simulink model "WischerBox"  (R2017b)
settings: Solver=FixedStepAuto  StartTime=0.0  StopTime=10.0  RelTol=1e-3
PreLoadFcn:
  | waijung.modelPreload; % Required for working with Waijung Blockset. Do not remove.
undefined symbols (not defined in the file): Blocking, HSEOSC, Link, LQFP100, Non, Raw, ST, STM32F407VG
libraries: simulink x16, stm32f4_canbus_lib x5, stm32f4_io_lib x2, stm32f4_adc_lib x1, stm32f4_device_config_lib x1
CloseFcn:
  | waijung.modelClose; % Required for working with Waijung Blockset. Do not remove.
settings Model: Creator=labuser  LastModifiedBy=labuser
settings OptimizationCC: DefaultParameterBehavior=Inlined  PassReuseOutputArgsAs=Individual arguments
settings DebuggingCC: ParameterTunabilityLossMsg=error
settings HardwareCC: ProdBitPerPointer=32  ProdBitPerSizeT=32  ProdBitPerPtrDiffT=32  ProdLargestAtomicFloat=None  ProdIntDivRoundTo=Undefined  ProdWordSize=32  ProdHWDeviceType=ARM Compatible->Cortex - M4  TargetEndianess=LittleEndian  TargetHWDeviceType=ARM Compatible->Cortex - M4
settings SFSimCC: MATLABDynamicMemAlloc=off
settings RTWCC: SystemTargetFile=stm32f4.tlc  GenerateMakefile=off  TemplateMakefile=ert_default_tmf  Description=STM32F4 Target  GenerateReport=on  IncludeHyperlinkInReport=on  LaunchReport=on  GenerateTraceInfo=on  GenerateTraceReport=on  GenerateTraceReportSl=on  GenerateTraceReportSf=on  GenerateTraceReportEml=on
settings CodeAppCC: ForceParamTrailComments=on  IgnoreCustomStorageClasses=off  OperatorAnnotations=on  SimulinkDataObjDesc=on  SFDataObjDesc=on  InsertBlockDesc=on
settings STFCustomTargetCC: TargetLangStandard=C99 (ISO)  MultiwordLength=256  ModelReferenceCompliant=off  CombineOutputUpdateFcns=on  ERTCustomFileBanners=on  SupportContinuousTime=off  SupportNonInlinedSFcns=off  RemoveResetFunc=on  MATLABClassNameForMDSCustomization=Simulink.SoftwareTarget.ERTCustomization  GRTInterface=off  SystemTargetFile=stm32f4.tlc
settings ERTTargetCC: TargetLangStandard=C99 (ISO)  ModelReferenceCompliant=off  ParMdlRefBuildCompliant=off  CompOptLevelCompliant=off  ConcurrentExecutionCompliant=off  ModelStepFunctionPrototypeControlCompliant=off  CPPClassGenCompliant=off  UseToolchainInfoCompliant=off  InlinedParameterPlacement=NonHierarchical  ERTSrcFileBannerTemplate=stm32f4_code_template.cgt  ERTHdrFileBannerTemplate=stm32f4_code_template.cgt  ERTDataSrcFileTemplate=stm32f4_code_template.cgt  ERTDataHdrFileTemplate=stm32f4_code_template.cgt  ERTCustomFileTemplate=stm32f4_file_process.tlc

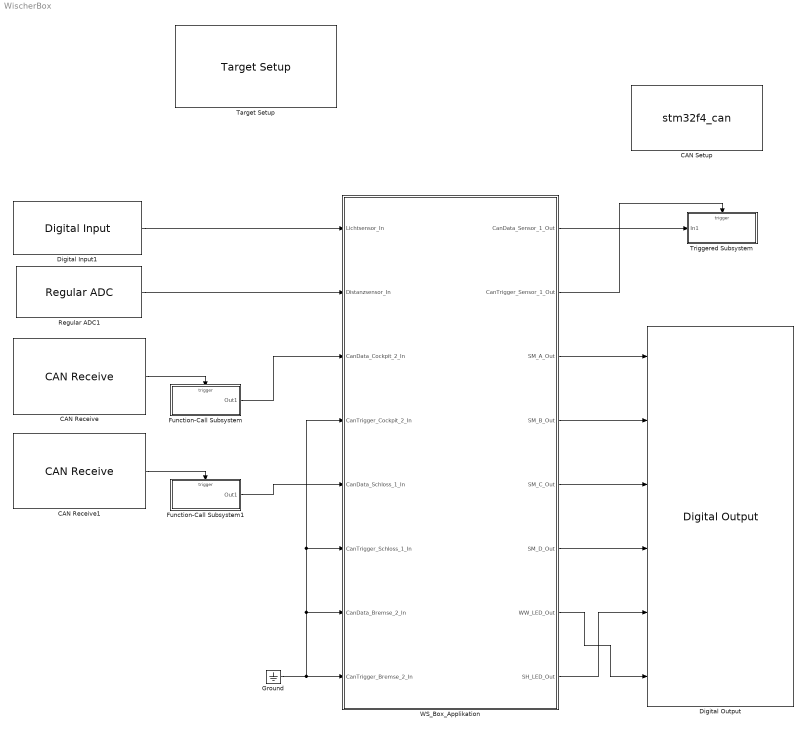
== system WischerBox ==
  CAN Receive : stm32f4_canbus_lib/CAN Receive  conf=Rx  canmodule=1  idtype=Standard  filtertype=Specific  id=17  idmask=0  enableisr=on  usedlc=off  datatype=single  data0type=uint32  data1type=uint32  data2type=Not used  data3type=Not used  data4type=Not used  data5type=Not used  data6type=Not used  data7type=Not used  buffersize=8  sampletime=-1  sampletimestr=-1  blockid=CANReceive  inputarray=[]  inputlabelarray={}  outputarray=[7]  outputlabelarray={'Call ISR' }  compat=0  confstr="[\"Standard\",\"Specific\",\"17\",\"0\",\"off\",\"uint32\",\"uint32\",\"Not used\",\"Not used\",\"Not used\",\"Not used\",\"Not used\",\"Not used\",\"8\",\"220\",\"0\",\"FFE0\",\"4\"]"
      settings: SourceProductName=Waijung Blockset
  CAN Receive1 : stm32f4_canbus_lib/CAN Receive  conf=Rx  canmodule=1  idtype=Standard  filtertype=Specific  id=25  idmask=0  enableisr=on  usedlc=off  datatype=single  data0type=uint32  data1type=uint32  data2type=Not used  data3type=Not used  data4type=Not used  data5type=Not used  data6type=Not used  data7type=Not used  buffersize=8  sampletime=-1  sampletimestr=-1  blockid=CANReceive1  inputarray=[]  inputlabelarray={}  outputarray=[7]  outputlabelarray={'Call ISR' }  compat=0  confstr="[\"Standard\",\"Specific\",\"25\",\"0\",\"off\",\"uint32\",\"uint32\",\"Not used\",\"Not used\",\"Not used\",\"Not used\",\"Not used\",\"Not used\",\"8\",\"320\",\"0\",\"FFE0\",\"4\"]"
      settings: SourceProductName=Waijung Blockset
  CAN Setup : S-Function  FunctionName=stm32f4_can  Parameters=conf,canmodule,0,inputarray,outputarray,'','',confstr,sampletime,sampletimestr,blockid  SFunctionDeploymentMode=off  EnableBusSupport=off  mask(stm32f4_can){conf=Setup, canmodule=1, advance=off, bitrate_select=125000, sjw=1tq, bs1=14tq, bs2=6tq, timingconf=Prescaler, brp=16, bitrate=125000, tq=3.8095e-07, autoretransmission=Disable, remaptxpin=D1, remaprxpin=D0, sampletime=0.01, sampletimestr=-1, blockid=CANSetup, inputarray=[], inputlabelarray={}, outputarray=[], outputlabelarray={}, compat=0, confstr=["125000","16","D","1","D","0","1tq","14tq","6tq","ENABLE"], presc=16, txportstr=D, txpinstr=1, rxportstr=D, rxpinstr=0, lastmodule=1}
      mask prompts: conf "Configuration"; canmodule "CAN Module"; advance "Advance configuration"; bitrate_select "Baud rate (bps)"; sjw "Resync Jump Width (SJW)"; bs1 "Bit segment 1 (BS1) + PROP_SEG"; bs2 "Bit segment 2 (BS2)"; timingconf "Adjust"; brp "Baud rate prescaler (BRP)"; bitrate "Baud rate (bps)"; tq "Time Quantum (Second), tq"; autoretransmission "Auto Re-transmission"; remaptxpin "CAN Tx pin"; remaprxpin "CAN Rx pin"; sampletime "Sample time (sec)"; sampletimestr "Compiled sample time (sec) in string"; inputarray "Input port"; inputlabelarray "Input port label"; outputarray "Output port"; outputlabelarray "Output port label"; compat "Compatibility (Reserved for future use)"; confstr "Configuration String"; presc "Prescale"; txportstr "Tx port string"; txpinstr "Tx pin string"; rxportstr "Rx port string"; rxpinstr "Rx pin string"; lastmodule "Last module selected"
      mask help:
      | This block setups CAN Module.
      |
      | Auto Re-transmission,
      |  - Enable: The CAN hardware will automatically retransmit the message until it has been
      | successfully transmitted according to the CAN standard.
      |  - Disable: A message will be transmitted only once, independently of the transmission result
      | (successful, error or arbitration lost).
      mask init:
      | stm32f4_can_callback('init');
      mask Help: web(fullfile(waijungdocroot,'stm32f4_can_setup.htm'), '-browser')
      mask TypeOptions conf: Setup
      mask TypeOptions canmodule: 1 | 2
      mask Callback canmodule: stm32f4_can_callback('canmodule');
      mask Callback advance: stm32f4_can_callback('advance');
      mask TypeOptions bitrate_select: 125000 | 250000 | 500000 | 1000000
      mask Callback bitrate_select: stm32f4_can_callback('bitrate_select');
      mask TypeOptions sjw: 1tq | 2tq | 3tq | 4tq
      mask TypeOptions bs1: 1tq | 2tq | 3tq | 4tq | 5tq | 6tq | 7tq | 8tq | 9tq | 10tq | 11tq | 12tq | 13tq | 14tq | 15tq | 16tq
      mask Callback bs1: stm32f4_can_callback('timingconf');
      mask TypeOptions bs2: 1tq | 2tq | 3tq | 4tq | 5tq | 6tq | 7tq | 8tq
      mask Callback bs2: stm32f4_can_callback('timingconf');
      mask TypeOptions timingconf: Prescaler | Baudrate
      mask Callback timingconf: stm32f4_can_callback('timingconf');
      mask Callback brp: stm32f4_can_callback('timingconf');
      mask Callback bitrate: stm32f4_can_callback('timingconf');
      mask TypeOptions autoretransmission: Enable | Disable
      mask TypeOptions remaptxpin: Not used | A12 | B9 | D1
      mask Callback remaptxpin: stm32f4_can_callback('remaptxpin');
      mask TypeOptions remaprxpin: Not used | A11 | B8 | D0
      mask Callback remaprxpin: stm32f4_can_callback('remaprxpin');
      mask Callback sampletime: stm32f4_can_callback('sampletime');
      mask Callback sampletimestr: stm32f4_can_callback('sampletimestr');
      mask Callback blockid: stm32f4_can_callback('blockid');
      mask Display: text(0.5, 0.5, 'CAN1_Setup\nSpeed (bps): 125000\nTx/Rx pin: D1/D0','ver','middle','hor','center');
  Digital Input1 : stm32f4_io_lib/Digital Input  port=C  speed=100  porttype=None  porttypestr=NOPULL  use_pin0=off  use_pin1=off  use_pin2=off  use_pin3=off  use_pin4=off  use_pin5=off  use_pin6=on  use_pin7=off  use_pin8=off  use_pin9=off  use_pin10=off  use_pin11=off  use_pin12=off  use_pin13=off  use_pin14=off  use_pin15=off  pinstr=GPIO_Pin_6  usedpinarray="[0  0  0  0  0  0  1  0  0  0  0  0  0  0  0  0]"  bitbandingstr="#define DigitalInput1_C6 Peripheral_BB(GPIOC->IDR, 6)  /* Output pin */"  sampletime=-1  sampletimestr=-1  blockid=DigitalInput1  enablecustomportlabel=off  glabalinit=off  cinputportlabel=In1, In2  coutputportlabel=Out1, Out2
      settings: SourceProductName=Waijung Blockset
  Digital Output : stm32f4_io_lib/Digital Output  use_bitband=on  port=C  speed=100  porttype=Push Pull  porttypestr=PP  use_pin0=on  use_pin1=on  use_pin2=on  use_pin3=on  use_pin4=on  use_pin5=on  use_pin6=off  use_pin7=off  use_pin8=off  use_pin9=off  use_pin10=off  use_pin11=off  use_pin12=off  use_pin13=off  use_pin14=off  use_pin15=off  pinstr=GPIO_Pin_0 | GPIO_Pin_1 | GPIO_Pin_2 | GPIO_Pin_3 | GPIO_Pin_4 | GPIO_Pin_5  usedpinarray="[1  1  1  1  1  1  0  0  0  0  0  0  0  0  0  0]"  bitbandingstr=|  sampletime=-1  sampletimestr=-1  blockid=DigitalOutput  enablecustomportlabel=off  globalinit=off  cinputportlabel=In1, In2  coutputportlabel=0
      | #define DigitalOutput_C0 Peripheral_BB(GPIOC->ODR, 0)  /* Output pin */
      | #define DigitalOutput_C1 Peripheral_BB(GPIOC->ODR, 1)  /* Output pin */
      | #define DigitalOutput_C2 Peripheral_BB(GPIOC->ODR, 2)  /* Output pin */
      | #define DigitalOutput_C3 Peripheral_BB(GPIOC->ODR, 3)  /* Output pin */
      | #define DigitalOutput_C4 Peripheral_BB(GPIOC->ODR, 4)  /* Output pin */
      | #define DigitalOutput_C5 Peripheral_BB(GPIOC->ODR, 5)  /* Output pin */
      settings: SourceProductName=Waijung Blockset
  Function-Call Subsystem : Subsystem  TreatAsAtomicUnit=on
  Function-Call Subsystem1 : Subsystem  TreatAsAtomicUnit=on
  Ground : Ground
  Regular ADC1 : stm32f4_adc_lib/Regular ADC  adcmodule=1  outputdatatype=Raw (uint16)  prescaler=2  prescalerstr=ADC_Prescaler_Div2  chsamplingtime=Auto  chsamplingtimestr=ADC_SampleTime_480Cycles  read_an0=on  read_an1=off  read_an2=off  read_an3=off  read_an4=off  read_an5=off  read_an6=off  read_an7=off  read_an8=off  read_an9=off  read_an10=off  read_an11=off  read_an12=off  read_an13=off  read_an14=off  read_an15=off  read_an16=off  read_an17=off  read_an18=off  pinstr=GPIO_Pin_0  usedpinarray="[1  0  0  0  0  0  0  0  0  0  0  0  0  0  0  0  0  0  0]"  usedportidarray=[0]  usedpinidarray=[0]  usedpinidcount=1  sampletime=-1  blockid=RegularADC1  enablecustomportlabel=off  cinputportlabel=0  coutputportlabel=Out1, Out2
      settings: SourceProductName=Waijung Blockset
  Target Setup : stm32f4_device_config_lib/Target Setup  Priority=100  compiler=GNU ARM  previous_compiler=GNU ARM  mcu=STM32F407VG (LQFP100)  mcustr=STM32F407VG  clockconfig=HSEOSC-8MHz  system_stm32f4xx_c_path=C:\waijung17_03a\targets\stm32f4_target\stm32f4\utils\system_stm32f4xx_default\STM32F40_41xxx\hseosc8mhz  showmemoryconfiguration=off  stacksize=0x2000  heapsize=0x2000  enableautocompiledownload=on  fullchiperase=off  programmerinterface=ST-Link  editctrlstr=on  compilercontrolstr=$(patsubst %, -I%, .) -mcpu=cortex-m4 -mthumb -mthumb-interwork -mfloat-abi=hard -mfpu=fpv4-sp-d16 -ffast-math -Wall -Wextra -Ofast  assemblercontrolstr=$(patsubst %, -I%, .) -mcpu=cortex-m4 -mthumb -mthumb-interwork -mfloat-abi=hard -mfpu=fpv4-sp-d16 -ffast-math -Wall -Wextra -Ofast -Wa,-amhls=$(<:.s=.lst) -D__STACK_SIZE=$(STACK_SIZE) -D__HEAP_SIZE=$(HEAP_SIZE)  linkercontrolstr=-T$(LD_SCRIPT) -g -Wl,-Map=$(MAP),--cref,--no-warn-mismatch -mcpu=cortex-m4 -mthumb -mthumb-interwork -mfloat-abi=hard -mfpu=fpv4-sp-d16 -specs=nosys.specs  runafterdownload=on  execprofile=None  profileruart=3  profilerbaud=500000  profilertxpin=D8  profilerinitstr=0.01,168000000,1680000,500000,0  manualsetsampletime=off  sampletime=0.01  blockid=TargetSetup  systickreloadvalue=1680000  hseval=8000000  lastprofileruart=3  hclk=168000000  flashorigin=0x8000000  flashlength=1024k  ramorigin=0x20000000  ramlength=128k  useextram=off
      settings: SourceProductName=Waijung Blockset
  Triggered Subsystem : Subsystem  TreatAsAtomicUnit=on
  WS_Box_Applikation : Subsystem
  wires:
  WS_Box_Applikation/8(SH_LED_Out) -> Digital Output/5
  Digital Input1/1 -> WS_Box_Applikation/1(Lichtsensor_In)
  WS_Box_Applikation/5(SM_C_Out) -> Digital Output/3
  Regular ADC1/1 -> WS_Box_Applikation/2(Distanzsensor_In)
  WS_Box_Applikation/3(SM_A_Out) -> Digital Output/1
  WS_Box_Applikation/6(SM_D_Out) -> Digital Output/4
  WS_Box_Applikation/7(WW_LED_Out) -> Digital Output/6
  WS_Box_Applikation/4(SM_B_Out) -> Digital Output/2
  CAN Receive1/1 -> Function-Call Subsystem1/Trigger
  WS_Box_Applikation/1(CanData_Sensor_1_Out) -> Triggered Subsystem/1(In1)
  Function-Call Subsystem1/1(Out1) -> WS_Box_Applikation/5(CanData_Schloss_1_In)
  CAN Receive/1 -> Function-Call Subsystem/Trigger
  WS_Box_Applikation/2(CanTrigger_Sensor_1_Out) -> Triggered Subsystem/Trigger
  Function-Call Subsystem/1(Out1) -> WS_Box_Applikation/3(CanData_Cockpit_2_In)
  Ground/1 -> WS_Box_Applikation/4(CanTrigger_Cockpit_2_In), WS_Box_Applikation/6(CanTrigger_Schloss_1_In), WS_Box_Applikation/7(CanData_Bremse_2_In), WS_Box_Applikation/8(CanTrigger_Bremse_2_In)

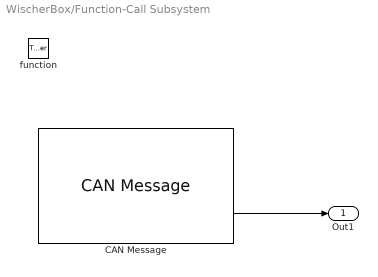
== system WischerBox/Function-Call Subsystem ==
  function : TriggerPort  TriggerType=function-call  VariantControl=Variant
  CAN Message : stm32f4_canbus_lib/CAN Message  conf=Msg  canmodule=1  usedlc=off  datatype=double  data0type=uint16  data1type=Not used  data2type=Not used  data3type=Not used  data4type=Not used  data5type=Not used  data6type=Not used  data7type=Not used  sampletime=-1  sampletimestr=-1  blockid=FunctionCallSubsystemCANMessage  inputarray=[]  inputlabelarray={}  outputarray=[ 7, 5]  outputlabelarray={'ID', 'D0 (uint16)' }  compat=0  confstr="[\"off\",\"uint16\",\"Not used\",\"Not used\",\"Not used\",\"Not used\",\"Not used\",\"Not used\",\"Not used\"]"
      settings: SourceProductName=Waijung Blockset
  Out1 : Outport
  wires:
  CAN Message/2 -> Out1/1

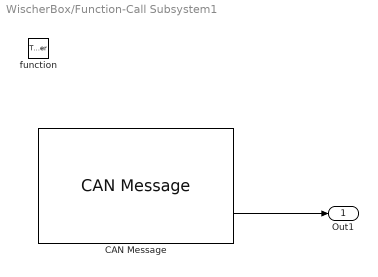
== system WischerBox/Function-Call Subsystem1 ==
  function : TriggerPort  TriggerType=function-call  VariantControl=Variant
  CAN Message : stm32f4_canbus_lib/CAN Message  conf=Msg  canmodule=1  usedlc=off  datatype=double  data0type=uint8  data1type=Not used  data2type=Not used  data3type=Not used  data4type=Not used  data5type=Not used  data6type=Not used  data7type=Not used  sampletime=-1  sampletimestr=-1  blockid=FunctionCallSubsystem1CANMessage  inputarray=[]  inputlabelarray={}  outputarray=[ 7, 3]  outputlabelarray={'ID', 'D0 (uint8)' }  compat=0  confstr="[\"off\",\"uint8\",\"Not used\",\"Not used\",\"Not used\",\"Not used\",\"Not used\",\"Not used\",\"Not used\"]"
      settings: SourceProductName=Waijung Blockset
  Out1 : Outport
  wires:
  CAN Message/2 -> Out1/1

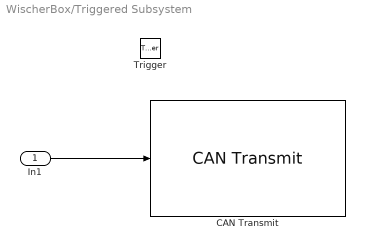
== system WischerBox/Triggered Subsystem ==
  In1 : Inport
  Trigger : TriggerPort  VariantControl=Variant
  CAN Transmit : stm32f4_canbus_lib/CAN Transmit  conf=Tx  canmodule=1  transfer=Non-Blocking  timeout=0.005  idtype=Standard  specificid=on  id=21  specificdlc=on  dlc=2  enablestatus=off  datatype=single  data0type=uint16  data1type=Not used  data2type=Not used  data3type=Not used  data4type=Not used  data5type=Not used  data6type=Not used  data7type=Not used  inputarray=[ 5]  inputlabelarray={ 'D0 (uint16)' }  outputarray=[]  outputlabelarray={}  sampletime=-1  sampletimestr=-1  blockid=TriggeredSubsystemCANTransmit  compat=0  confstr="[\"Non-Blocking\",\"0.005\",\"Standard\",\"on\",\"21\",\"on\",\"2\",\"off\",\"uint16\",\"Not used\",\"Not used\",\"Not used\",\"Not used\",\"Not used\",\"Not used\",\"Not used\"]"
      settings: SourceProductName=Waijung Blockset
  wires:
  In1/1 -> CAN Transmit/1

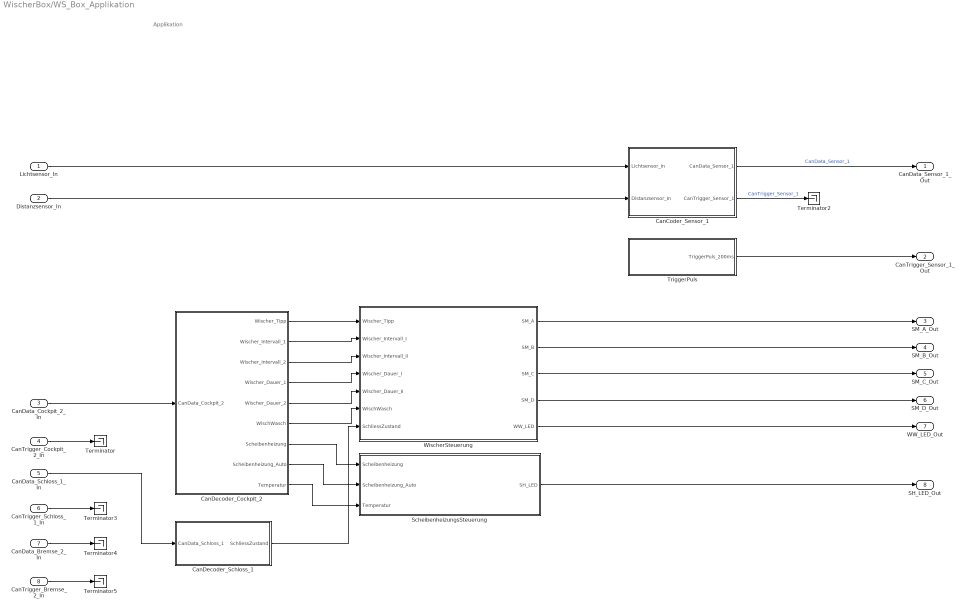
== system WischerBox/WS_Box_Applikation ==
  note: Applikation
  Lichtsensor_In : Inport
  Distanzsensor_In : Inport  Port=2
  CanData_Cockpit_2_In : Inport  Port=3
  CanTrigger_Cockpit_2_In : Inport  Port=4
  CanData_Schloss_1_In : Inport  Port=5
  CanTrigger_Schloss_1_In : Inport  Port=6
  CanData_Bremse_2_In : Inport  Port=7
  CanTrigger_Bremse_2_In : Inport  Port=8
  CanCoder_Sensor_1 : Subsystem
  CanDecoder_Cockpit_2 : Subsystem
  CanDecoder_Schloss_1 : Subsystem
  ScheibenheizungsSteuerung : Stateflow chart  TreatAsAtomicUnit=on
  Terminator{,2..5} (5 alike) : Terminator
  TriggerPuls : Subsystem
  WischerSteuerung : Stateflow chart  TreatAsAtomicUnit=on
  CanData_Sensor_1_Out : Outport
  CanTrigger_Sensor_1_Out : Outport  Port=2
  SM_A_Out : Outport  Port=3
  SM_B_Out : Outport  Port=4
  SM_C_Out : Outport  Port=5
  SM_D_Out : Outport  Port=6
  WW_LED_Out : Outport  Port=7
  SH_LED_Out : Outport  Port=8
  wires:
  ScheibenheizungsSteuerung/1(SH_LED) -> SH_LED_Out/1
  WischerSteuerung/3(SM_C) -> SM_C_Out/1
  WischerSteuerung/5(WW_LED) -> WW_LED_Out/1
  CanCoder_Sensor_1/1(CanData_Sensor_1) -> CanData_Sensor_1_Out/1  "CanData_Sensor_1"
  WischerSteuerung/1(SM_A) -> SM_A_Out/1
  WischerSteuerung/4(SM_D) -> SM_D_Out/1
  WischerSteuerung/2(SM_B) -> SM_B_Out/1
  TriggerPuls/1(TriggerPuls_200ms) -> CanTrigger_Sensor_1_Out/1
  Distanzsensor_In/1 -> CanCoder_Sensor_1/2(Distanzsensor_In)
  Lichtsensor_In/1 -> CanCoder_Sensor_1/1(Lichtsensor_In)
  CanData_Schloss_1_In/1 -> CanDecoder_Schloss_1/1(CanData_Schloss_1)
  CanTrigger_Cockpit_2_In/1 -> Terminator/1
  CanData_Cockpit_2_In/1 -> CanDecoder_Cockpit_2/1(CanData_Cockpit_2)
  CanDecoder_Cockpit_2/3(Wischer_Intervall_2) -> WischerSteuerung/3(Wischer_Intervall_II)
  CanDecoder_Cockpit_2/9(Temperatur) -> ScheibenheizungsSteuerung/3(Temperatur)
  CanDecoder_Cockpit_2/8(Scheibenheizung_Auto) -> ScheibenheizungsSteuerung/2(Scheibenheizung_Auto)
  CanDecoder_Cockpit_2/7(Scheibenheizung) -> ScheibenheizungsSteuerung/1(Scheibenheizung)
  CanDecoder_Cockpit_2/2(Wischer_Intervall_1) -> WischerSteuerung/2(Wischer_Intervall_I)
  CanDecoder_Cockpit_2/1(Wischer_Tipp) -> WischerSteuerung/1(Wischer_Tipp)
  CanDecoder_Cockpit_2/4(Wischer_Dauer_1) -> WischerSteuerung/4(Wischer_Dauer_I)
  CanDecoder_Cockpit_2/5(Wischer_Dauer_2) -> WischerSteuerung/5(Wischer_Dauer_II)
  CanDecoder_Cockpit_2/6(WischWasch) -> WischerSteuerung/6(WischWasch)
  CanTrigger_Bremse_2_In/1 -> Terminator5/1
  CanData_Bremse_2_In/1 -> Terminator4/1
  CanTrigger_Schloss_1_In/1 -> Terminator3/1
  CanCoder_Sensor_1/2(CanTrigger_Sensor_1) -> Terminator2/1  "CanTrigger_Sensor_1"
  CanDecoder_Schloss_1/1(SchliessZustand) -> WischerSteuerung/7(SchliessZustand)

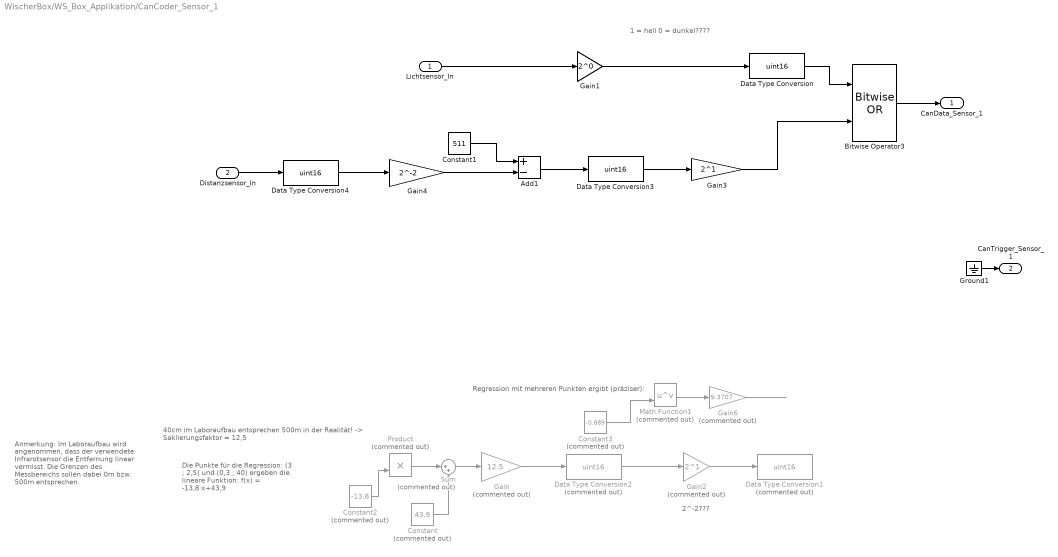
== system WischerBox/WS_Box_Applikation/CanCoder_Sensor_1 ==
  note: 1 = hell
      | 0 = dunkel????
  note: Regression mit mehreren Punkten ergibt (präziser):
  note: Die Punkte für die Regression:
      | (3 ; 2,5) und (0,3 ; 40)
      |
      | ergeben die lineare Funktion:
      | f(x) = -13,8·x+43,9
  note: Anmerkung: Im Laboraufbau wird angenommen, dass der verwendete Infrarotsensor die Entfernung linear vermisst. Die Grenzen des Messbereichs sollen dabei 0m bzw. 500m entsprechen.
  note: 40cm im Laboraufbau entsprechen 500m in der Realität!
      | -> Saklierungsfaktor = 12,5
  note: 2^-2???
  Lichtsensor_In : Inport
  Distanzsensor_In : Inport  Port=2
  Add1 : Sum  Inputs=+-
  Bitwise Operator3 : simulink/Logic and Bit Operations/Bitwise Operator  logicop=OR  UseBitMask=off  NumInputPorts=2  BitMask=bin2dec('11011001')  BitMaskRealWorld=Stored Integer
  Constant : Constant  Commented=on  Value=43.9
  Constant1 : Constant  Value=511
  Constant2 : Constant  Commented=on  Value=-13.8
  Constant3 : Constant  Commented=on  Value=-0.889
  Data Type Conversion : DataTypeConversion  OutDataTypeStr=uint16
  Data Type Conversion1 : DataTypeConversion  Commented=on  OutDataTypeStr=uint16
  Data Type Conversion2 : DataTypeConversion  Commented=on  OutDataTypeStr=uint16
  Data Type Conversion3 : DataTypeConversion  OutDataTypeStr=uint16
  Data Type Conversion4 : DataTypeConversion  OutDataTypeStr=uint16
  Gain : Gain  Commented=on  Gain=12.5
  Gain1 : Gain  Gain=2^0
  Gain2 : Gain  Commented=on  Gain=2^1
  Gain3 : Gain  Gain=2^1  ParamDataTypeStr=uint16  OutDataTypeStr=uint16
  Gain4 : Gain  Gain=2^-2
  Gain6 : Gain  Commented=on  Gain=9.3707
  Ground1 : Ground
  Math Function1 : Math  Commented=on  Operator=pow  SaturateOnIntegerOverflow=on
  Product : Product  Commented=on
  Sum : Sum  Commented=on  Inputs=|++
  CanData_Sensor_1 : Outport
  CanTrigger_Sensor_1 : Outport  Port=2
  wires:
  Ground1/1 -> CanTrigger_Sensor_1/1
  Bitwise Operator3/1 -> CanData_Sensor_1/1
  Gain1/1 -> Data Type Conversion/1
  Data Type Conversion/1 -> Bitwise Operator3/1
  Sum/1 -> Gain/1
  Gain6/1 -> ?
  Constant3/1 -> Math Function1/2
  Math Function1/1 -> Gain6/1
  Constant2/1 -> Product/2
  Constant/1 -> Sum/2
  Product/1 -> Sum/1
  Lichtsensor_In/1 -> Gain1/1
  Gain2/1 -> Data Type Conversion1/1
  Gain/1 -> Data Type Conversion2/1
  Data Type Conversion2/1 -> Gain2/1
  Data Type Conversion4/1 -> Gain4/1
  Data Type Conversion3/1 -> Gain3/1
  Add1/1 -> Data Type Conversion3/1
  Constant1/1 -> Add1/1
  Gain4/1 -> Add1/2
  Gain3/1 -> Bitwise Operator3/2
  Distanzsensor_In/1 -> Data Type Conversion4/1

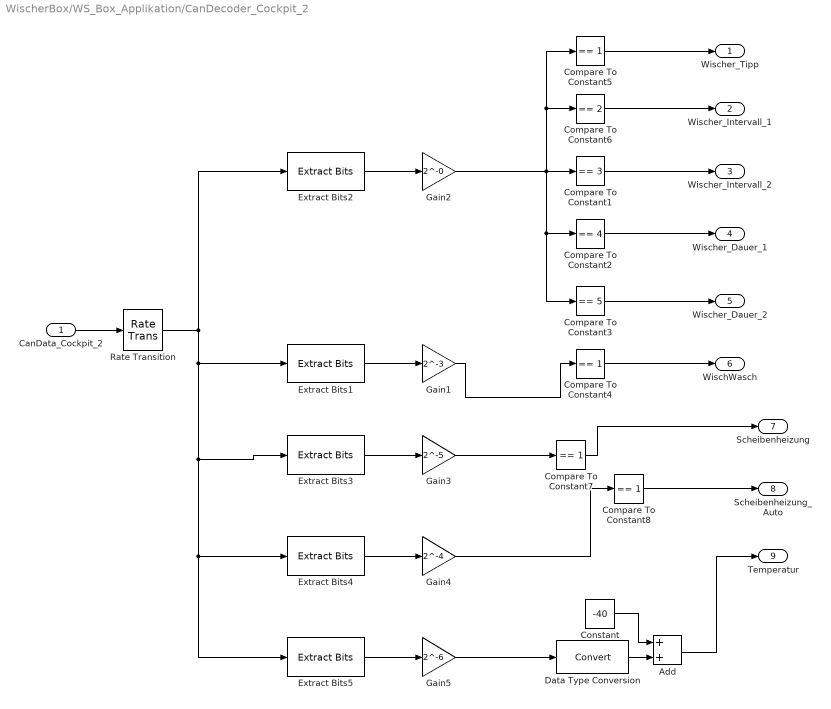
== system WischerBox/WS_Box_Applikation/CanDecoder_Cockpit_2 ==
  CanData_Cockpit_2 : Inport
  Add : Sum
  Compare To Constant1 : simulink/Logic and Bit Operations/Compare To Constant  relop===  const=3  OutDataTypeStr=boolean
  Compare To Constant2 : simulink/Logic and Bit Operations/Compare To Constant  relop===  const=4  OutDataTypeStr=boolean
  Compare To Constant3 : simulink/Logic and Bit Operations/Compare To Constant  relop===  const=5  OutDataTypeStr=boolean
  Compare To Constant{4..5,7..8} (4 alike) : simulink/Logic and Bit Operations/Compare To Constant  relop===  const=1  OutDataTypeStr=boolean
  Compare To Constant6 : simulink/Logic and Bit Operations/Compare To Constant  relop===  const=2  OutDataTypeStr=boolean
  Constant : Constant  Value=-40
  Data Type Conversion : DataTypeConversion  RndMeth=Zero
  Extract Bits1 : simulink/Logic and Bit Operations/Extract Bits  bitsToExtract=Range of bits  numBits=8  bitIdxRange=3  outScalingMode=Preserve fixed-point scaling
  Extract Bits2 : simulink/Logic and Bit Operations/Extract Bits  bitsToExtract=Range of bits  numBits=8  bitIdxRange=[0 2]  outScalingMode=Preserve fixed-point scaling
  Extract Bits3 : simulink/Logic and Bit Operations/Extract Bits  bitsToExtract=Range of bits  numBits=8  bitIdxRange=5  outScalingMode=Preserve fixed-point scaling
  Extract Bits4 : simulink/Logic and Bit Operations/Extract Bits  bitsToExtract=Range of bits  numBits=8  bitIdxRange=4  outScalingMode=Preserve fixed-point scaling
  Extract Bits5 : simulink/Logic and Bit Operations/Extract Bits  bitsToExtract=Range of bits  numBits=8  bitIdxRange=[6 12]  outScalingMode=Preserve fixed-point scaling
  Gain1 : Gain  Gain=2^-3
  Gain2 : Gain  Gain=2^-0
  Gain3 : Gain  Gain=2^-5
  Gain4 : Gain  Gain=2^-4
  Gain5 : Gain  Gain=2^-6
  Rate Transition : RateTransition  Deterministic=off  OutPortSampleTimeOpt=Inherit
  Wischer_Tipp : Outport
  Wischer_Intervall_1 : Outport  Port=2
  Wischer_Intervall_2 : Outport  Port=3
  Wischer_Dauer_1 : Outport  Port=4
  Wischer_Dauer_2 : Outport  Port=5
  WischWasch : Outport  Port=6
  Scheibenheizung : Outport  Port=7
  Scheibenheizung_Auto : Outport  Port=8
  Temperatur : Outport  Port=9
  wires:
  CanData_Cockpit_2/1 -> Rate Transition/1
  Gain4/1 -> Compare To Constant8/1
  Gain3/1 -> Compare To Constant7/1
  Data Type Conversion/1 -> Add/2
  Gain2/1 -> Compare To Constant2/1, Compare To Constant3/1, Compare To Constant1/1, Compare To Constant6/1, Compare To Constant5/1
  Extract Bits2/1 -> Gain2/1
  Compare To Constant3/1 -> Wischer_Dauer_2/1
  Compare To Constant2/1 -> Wischer_Dauer_1/1
  Compare To Constant1/1 -> Wischer_Intervall_2/1
  Compare To Constant6/1 -> Wischer_Intervall_1/1
  Compare To Constant5/1 -> Wischer_Tipp/1
  Extract Bits1/1 -> Gain1/1
  Extract Bits3/1 -> Gain3/1
  Compare To Constant7/1 -> Scheibenheizung/1
  Extract Bits4/1 -> Gain4/1
  Compare To Constant8/1 -> Scheibenheizung_Auto/1
  Extract Bits5/1 -> Gain5/1
  Gain5/1 -> Data Type Conversion/1
  Add/1 -> Temperatur/1
  Constant/1 -> Add/1
  Rate Transition/1 -> Extract Bits2/1, Extract Bits1/1, Extract Bits5/1, Extract Bits4/1, Extract Bits3/1
  Compare To Constant4/1 -> WischWasch/1
  Gain1/1 -> Compare To Constant4/1

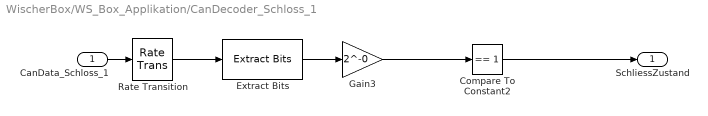
== system WischerBox/WS_Box_Applikation/CanDecoder_Schloss_1 ==
  CanData_Schloss_1 : Inport
  Compare To Constant2 : simulink/Logic and Bit Operations/Compare To Constant  relop===  const=1  OutDataTypeStr=boolean
  Extract Bits : simulink/Logic and Bit Operations/Extract Bits  bitsToExtract=Range of bits  numBits=8  bitIdxRange=[0]  outScalingMode=Preserve fixed-point scaling
  Gain3 : Gain  Gain=2^-0  OutDataTypeStr=uint8
  Rate Transition : RateTransition  Deterministic=off  OutPortSampleTimeOpt=Inherit
  SchliessZustand : Outport
  wires:
  Gain3/1 -> Compare To Constant2/1
  Extract Bits/1 -> Gain3/1
  CanData_Schloss_1/1 -> Rate Transition/1
  Rate Transition/1 -> Extract Bits/1
  Compare To Constant2/1 -> SchliessZustand/1

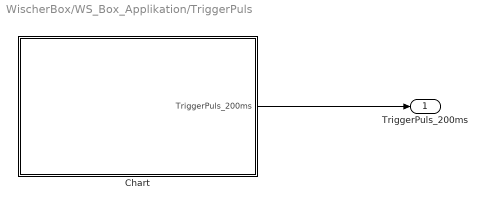
== system WischerBox/WS_Box_Applikation/TriggerPuls ==
  Chart : Stateflow chart  TreatAsAtomicUnit=on
  TriggerPuls_200ms : Outport
  wires:
  Chart/1(TriggerPuls_200ms) -> TriggerPuls_200ms/1

== stateflow chart WischerBox/WS_Box_Applikation/WischerSteuerung ==
  state Wischer_AUS
    entry:
    WW_LED=false;
    SM_A=false;
    SM_B=false;
    SM_C=false;
    SM_D=false;
  state Spruehen
    entry:
    WW_LED=true;
    WW_Mode=true;
  state Wischer_AN
    state Wischbewegung [parallel]
      entry:
      SM_A=false;
      SM_B=false;
      SM_C=false;
      SM_D=false;
      Step=0;
      Count=0;
      settings: executionOrder=2
      state Dauertippen
      state Hinwueschen
        state A
          entry:
          SM_A=true;
          SM_B=false;
          SM_C=false;
          SM_D=false;
        state B
          entry:
          SM_A=false;
          SM_B=true;
          SM_C=false;
          SM_D=false;
        state D
          entry:
          SM_A=false;
          SM_B=false;
          SM_C=false;
          SM_D=true;
        state C
          entry:
          SM_A=false;
          SM_B=false;
          SM_C=true;
          SM_D=false;
        (default) -> Wischer_AN.Wischbewegung.Hinwueschen.A : {Count=Count+1}
        Wischer_AN.Wischbewegung.Hinwueschen.A -> Wischer_AN.Wischbewegung.Hinwueschen.B : after(delay,sec){Step=Step+1}
        Wischer_AN.Wischbewegung.Hinwueschen.D -> Wischer_AN.Wischbewegung.Hinwueschen.A : after(delay,sec){Step=Step+1}
        Wischer_AN.Wischbewegung.Hinwueschen.B -> Wischer_AN.Wischbewegung.Hinwueschen.C : after(delay,sec){Step=Step+1}
        Wischer_AN.Wischbewegung.Hinwueschen.C -> Wischer_AN.Wischbewegung.Hinwueschen.D : after(delay,sec){Step=Step+1}
      state Zurueckwueschen
        state A
          entry:
          SM_A=true;
          SM_B=false;
          SM_C=false;
          SM_D=false;
        state B
          entry:
          SM_A=false;
          SM_B=true;
          SM_C=false;
          SM_D=false;
        state D
          entry:
          SM_A=false;
          SM_B=false;
          SM_C=false;
          SM_D=true;
        state C
          entry:
          SM_A=false;
          SM_B=false;
          SM_C=true;
          SM_D=false;
        (default) -> Wischer_AN.Wischbewegung.Zurueckwueschen.A
        Wischer_AN.Wischbewegung.Zurueckwueschen.B -> Wischer_AN.Wischbewegung.Zurueckwueschen.A : after(delay,sec){Step=Step-1}
        Wischer_AN.Wischbewegung.Zurueckwueschen.A -> Wischer_AN.Wischbewegung.Zurueckwueschen.D : after(delay,sec){Step=Step-1}
        Wischer_AN.Wischbewegung.Zurueckwueschen.C -> Wischer_AN.Wischbewegung.Zurueckwueschen.B : after(delay,sec){Step=Step-1}
        Wischer_AN.Wischbewegung.Zurueckwueschen.D -> Wischer_AN.Wischbewegung.Zurueckwueschen.C : after(delay,sec){Step=Step-1}
      state vier_s
      state zwei_s
      state WARTEN
      Dauertippen -> Hinwueschen : [stop==false]
      Zurueckwueschen -> Dauertippen [order 1] : [Step==0 && stop==true]
      (default) -> Hinwueschen
      Hinwueschen -> Zurueckwueschen : [Step==20]
      Zurueckwueschen -> WARTEN [order 2] : [Step==0]
      vier_s -> Hinwueschen : after(4,sec)
      zwei_s -> Hinwueschen : after(2,sec)
      WARTEN -> Hinwueschen [order 1] : [Wischer_Intervall_I==0 && Wischer_Intervall_II==0]
      WARTEN -> vier_s [order 2] : [Wischer_Intervall_I==1]
      WARTEN -> zwei_s [order 3] : [Wischer_Intervall_II==1]
    state Wischsteuerung [parallel]
      settings: executionOrder=1
      state Wischerstellung
        entry:
        stop=false;
      state Tippzustand
        entry:
        stop=true;
      state WischWasch
        entry:
        pause=0;
        wischen=2;
        delay=(wischen/40);
        Count=0;
      state Wischer_Tipp
        entry:
        pause=4;
        wischen=2;
        delay=(wischen/40);
        Count=0;
      state Wischer_Intervall_I
        entry:
        pause=4;
        wischen=2;
        delay=(wischen/40);
        Count=1;
      state Wischer_Intervall_II
        entry:
        pause=2;
        wischen=2;
        delay=(wischen/40);
        Count=1;
      state Wischer_Dauer_I
        entry:
        pause=0;
        wischen=2;
        delay=(wischen/40);
        Count=0;
      state Wischer_Dauer_II
        entry:
        pause=0;
        wischen=1;
        delay=(wischen/40);
        Count=0;
      (default) -> Wischerstellung
      Wischerstellung -> WischWasch [order 6] : [WW_Mode==true]
      Wischerstellung -> Wischer_Tipp [order 2] : [Wischer_Tipp==1]
      Tippzustand -> Wischerstellung : [Wischer_Tipp==0]
      Wischerstellung -> Wischer_Intervall_I [order 4] : [Wischer_Intervall_I==1]
      Wischer_Intervall_I -> Wischerstellung : [Wischer_Intervall_I==0 && Step==0]
      Wischerstellung -> Wischer_Intervall_II [order 5] : [Wischer_Intervall_II==1]
      Wischer_Intervall_II -> Wischerstellung : [Wischer_Intervall_II==0 && Step==0]
      Wischerstellung -> Wischer_Dauer_I [order 3] : [Wischer_Dauer_I==1]
      Wischer_Dauer_I -> Wischerstellung : [Wischer_Tipp==0 && Step==0]
      Wischerstellung -> Wischer_Dauer_II [order 1] : [Wischer_Dauer_II==1]
      Wischer_Dauer_II -> Wischerstellung : [Wischer_Dauer_II==0 && Step==0]
      Wischer_Tipp -> Tippzustand
    state Spruehen [parallel]
      settings: executionOrder=3
      state OFF
        entry:
        WW_LED=false;
      state ON
        entry:
        WW_LED=true;
      (default) -> OFF
      OFF -> ON : [WischWasch==1 && SchliessZustand==1]
      ON -> OFF : after(2, sec)
  (default) -> Wischer_AUS : {WW_Mode=false}
  Wischer_AUS -> Spruehen [order 2] : [WischWasch==1 && SchliessZustand==1]
  Spruehen -> Wischer_AUS : after(2, sec)
  Wischer_AUS -> Wischer_AN [order 1] : [Wischer_Tipp==1 || Wischer_Intervall_I==1 || Wischer_Intervall_II==1 || Wischer_Dauer_I==1 || Wischer_Dauer_II==1]
  Wischer_AN -> Wischer_AUS [order 1] : [Wischer_Tipp==0 && Wischer_Intervall_I==0 && Wischer_Intervall_II==0 && Wischer_Dauer_I==0 && Wischer_Dauer_II==0 && Step==0 && WW_Mode==false]
  Wischer_AUS -> Wischer_AN [order 3] : [WW_Mode==true]
  Wischer_AN -> Wischer_AUS [order 2] : [Count==3 && WW_Mode==true]{WW_Mode=false}
  data: Wischer_Tipp input; Wischer_Intervall_I input; Wischer_Intervall_II input; Wischer_Dauer_I input; Wischer_Dauer_II input; WischWasch input; SM_A output; SM_B output; SM_C output; SM_D output; WW_LED output; Step local uint16; Forward local; StepTime local; StepTime1 local; Count local int16; wisher_delay local double; wisher_cnt local uint8; wisher_dir local boolean; wisher_active local boolean; wisher_timeout local double; SchliessZustand input; delay local double; wischen local double; dauer local int16; pause local int8; data local; WW_Mode local boolean; stop local boolean

== stateflow chart WischerBox/WS_Box_Applikation/ScheibenheizungsSteuerung ==
  state STEUERUNG [parallel]
    settings: executionOrder=2
    state MANUELL
      entry:
      Heizen=false;
      state AN
        entry:
        Heizen=true;
      state AUS
        entry:
        Heizen=false;
      state DEAKTIVIERT
        entry:
        Heizen=false;
      (default) -> STEUERUNG.MANUELL.AUS
      STEUERUNG.MANUELL.AUS -> STEUERUNG.MANUELL.AN : [Scheibenheizung==1]
      STEUERUNG.MANUELL.AN -> STEUERUNG.MANUELL.DEAKTIVIERT [order 2] : after(30,sec)
      STEUERUNG.MANUELL.DEAKTIVIERT -> STEUERUNG.MANUELL.AUS : [Scheibenheizung==0]
      STEUERUNG.MANUELL.AN -> STEUERUNG.MANUELL.DEAKTIVIERT [order 1] : [Scheibenheizung==0]
    state AUTOMATIK
      entry:
      Heizen=false;
      state AN
        entry:
        Heizen=true;
      state AUS
        entry:
        Heizen=false;
      state DEAKTIVIERT
        entry:
        Heizen=false;
      (default) -> STEUERUNG.AUTOMATIK.AUS
      STEUERUNG.AUTOMATIK.AUS -> STEUERUNG.AUTOMATIK.AN : [Temperatur<2]
      STEUERUNG.AUTOMATIK.AN -> STEUERUNG.AUTOMATIK.DEAKTIVIERT [order 2] : after(30,sec)
      STEUERUNG.AUTOMATIK.DEAKTIVIERT -> STEUERUNG.AUTOMATIK.AUS [order 2] : [Temperatur>=2]
      STEUERUNG.AUTOMATIK.AN -> STEUERUNG.AUTOMATIK.DEAKTIVIERT [order 1] : [Temperatur>=2]
      STEUERUNG.AUTOMATIK.DEAKTIVIERT -> STEUERUNG.AUTOMATIK.AUS [order 1] : [Scheibenheizung_Auto==0]
      STEUERUNG.AUTOMATIK.AN -> STEUERUNG.AUTOMATIK.DEAKTIVIERT [order 3] : [Scheibenheizung_Auto==0]
    (default) -> MANUELL
    MANUELL -> AUTOMATIK : [Scheibenheizung_Auto==1]
    AUTOMATIK -> MANUELL : [Scheibenheizung_Auto==0]
  state SCHEIBENHEIZUNG [parallel]
    entry:
    SH_LED=false;
    settings: executionOrder=1
    state AUS
      entry:
      SH_LED=false;
    state AN
      entry:
      SH_LED=true;
    state warten_bei_AUTO
    state AUS_bis_Neustart
      entry:
      SH_LED=false;
    state AN_nur_Manuell
      entry:
      SH_LED=true;
    (default) -> SCHEIBENHEIZUNG.AUS
    SCHEIBENHEIZUNG.AUS -> SCHEIBENHEIZUNG.AN : [Heizen==true]
    SCHEIBENHEIZUNG.AN -> SCHEIBENHEIZUNG.AUS [order 1] : [Heizen==false]
    SCHEIBENHEIZUNG.AN -> warten_bei_AUTO [order 2] : [Scheibenheizung_Auto==1]
    warten_bei_AUTO -> AUS_bis_Neustart : after(30,sec)
    AUS_bis_Neustart -> AN_nur_Manuell : [Scheibenheizung_Auto==0 && Heizen==true]
    AN_nur_Manuell -> AUS_bis_Neustart : [Heizen==false]
  data: Scheibenheizung input; Scheibenheizung_Auto input; Temperatur input; SH_LED output; Heizen local boolean

== stateflow chart WischerBox/WS_Box_Applikation/TriggerPuls/Chart ==
  state Off
    en, du: TriggerPuls_200ms = 0;
  state On
    en, du: TriggerPuls_200ms = 1;
  (default) -> On
  On -> Off : after(0.5,sec)
  Off -> On : after(0.5,sec)
  data: TriggerPuls_200ms output
